simulink model "Regler"  (R2021b)
settings: Solver=ode23s  StartTime=tSim(1)  StopTime=tSim(end)  FixedStep=tStep  RelTol=1e-3  EnableMultiTasking=on
values from neighbouring files (symbols this model uses):
  k_Position = 6.92    [reglerInit.m]
settings Model: Creator=Henning Schlüter  LastModifiedBy=liams
settings SolverCC: AlgebraicLoopSolver=TrustRegion
settings DataIOCC: SaveFormat=Array  SignalLoggingSaveFormat=ModelDataLogs  SaveOutput=off  SaveTime=off  ReturnWorkspaceOutputs=off
settings OptimizationCC: ExpressionDepthLimit=2147483647  LifeSpan=inf
settings DebuggingCC: UnderspecifiedInitializationDetection=Classic  MergeDetectMultiDrivingBlocksExec=none  SolverPrmCheckMsg=warning  StateNameClashWarn=warning  PregeneratedLibrarySubsystemCodeDiagnostic=none  SFUnexpectedBacktrackingDiag=warning  SFNoUnconditionalDefaultTransitionDiag=warning  SFExecutionAtInitializationDiag=none  SFMachineParentedDataDiag=warning  ArithmeticOperatorsInVariantConditions=warning
settings HardwareCC: ProdBitPerPointer=32  ProdBitPerSizeT=32  ProdBitPerPtrDiffT=32  ProdLargestAtomicFloat=None  ProdIntDivRoundTo=Undefined  ProdEndianess=Unspecified  ProdWordSize=32  ProdHWDeviceType=32-bit Generic
settings ModelReferenceCC: PropagateSignalLabelsOutOfModel=off
settings SFSimCC: SimUseLocalCustomCode=off  CustomCodeUndefinedFunction=UseInterfaceOnly
settings RTWCC: RTWUseLocalCustomCode=off
settings CodeAppCC: StateflowObjectComments=on
settings GRTTargetCC: TargetLangStandard=C89/C90 (ANSI)  CombineOutputUpdateFcns=off  GRTInterface=on
settings ConfigComp: CovMetricSettings=dw  CovSaveCumulativeToWorkspaceVar=on  CovSaveSingleToWorkspaceVar=on  CovExternalEMLEnable=off  CovSFcnEnable=off

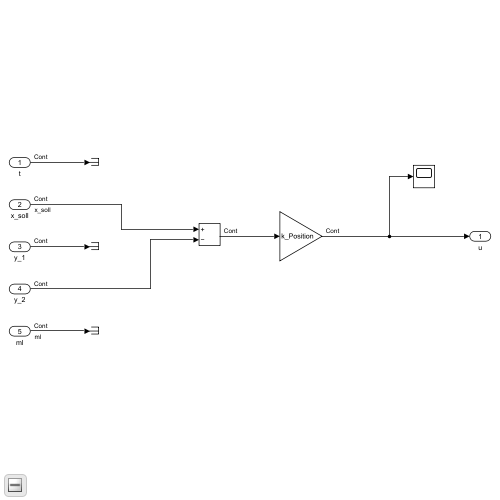
[thumbnail: Simulink's stored preview of the top-level diagram]
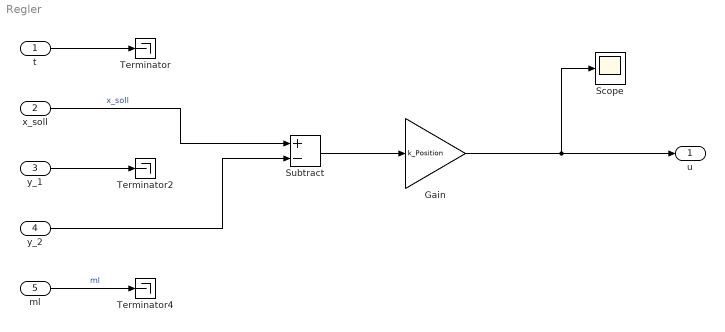
== system Regler ==
  t : Inport  OutDataTypeStr=double  PortDimensions=1  SampleTime=0
  "x_soll " : Inport  Port=2  OutDataTypeStr=double  PortDimensions=1  SampleTime=0
  y_1 : Inport  Port=3  OutDataTypeStr=double  PortDimensions=[1 1]  SampleTime=0
  y_2 : Inport  Port=4  OutDataTypeStr=double  PortDimensions=[1 1]  SampleTime=0
  ml : Inport  Port=5  OutDataTypeStr=double  PortDimensions=1  SampleTime=0
  Gain : Gain  Gain=k_Position
  Scope : Scope
  Subtract : Sum  Inputs=+-
  Terminator : Terminator
  Terminator2 : Terminator
  Terminator4 : Terminator
  u : Outport  OutDataTypeStr=double  PortDimensions=1  VectorParamsAs1DForOutWhenUnconnected=off
  wires:
  t/1 -> Terminator/1
  "x_soll "/1 -> Subtract/1  "x_soll"
  y_1/1 -> Terminator2/1
  ml/1 -> Terminator4/1  "ml"
  Gain/1 -> Scope/1, u/1
  y_2/1 -> Subtract/2
  Subtract/1 -> Gain/1
